simulink model "sampleModel548_pp_difftest"  (R2021a)
settings: Solver=VariableStepAuto  StartTime=0.0  StopTime=10.0  RelTol=1e-3
undefined symbols (not defined in the file or in its folder): DiscIntNeverNeededParam, Newton, Raphson
libraries: simulink x55, pid_lib x8
(part 2 of 2)

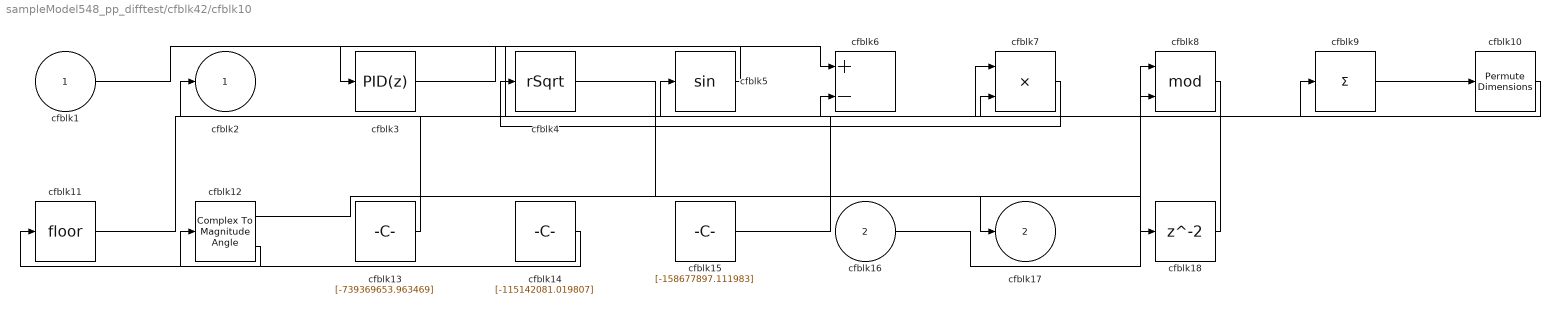
== system sampleModel548_pp_difftest/cfblk42/cfblk10 ==
  cfblk1 : Inport
  cfblk16 : Inport  Port=2
  cfblk10 : PermuteDimensions
  cfblk11 : Rounding
  cfblk12 : ComplexToMagnitudeAngle
  cfblk13 : Constant  Value=[-739369653.963469]  SampleTime=1
  cfblk14 : Constant  Value=[-115142081.019807]  SampleTime=1
  cfblk15 : Constant  Value=[-158677897.111983]  SampleTime=1
  cfblk18 : Delay  SampleTime=1
  cfblk3 : pid_lib/PID Controller  Controller=PID  Form=Parallel  TimeDomain=Discrete-time  UseExternalTs=off  SampleTime=1  IntegratorMethod=Forward Euler  FilterMethod=Forward Euler  ControllerParametersSource=internal  P=1  I=1  D=0  UseFilter=on  N=100  TunerSelectOption=Transfer Function Based (PID Tuner App)  InitialConditionSource=internal  InitialConditionForIntegrator=0  InitialConditionForFilter=0  DifferentiatorICPrevScaledInput=0  ExternalReset=none  TrackingMode=off  Kt=1  LimitOutput=off  SatLimitsSource=internal  UpperSaturationLimit=inf  LowerSaturationLimit=-inf  LinearizeAsGain=off  AntiWindupMode=none  Kb=1  POutMin=[]  POutMax=[]  IOutMin=[]  IOutMax=[]  DOutMin=[]  DOutMax=[]  NOutMin=[]  NOutMax=[]  SumOutMin=[]  SumOutMax=[]  SaturationOutMin=[]  SaturationOutMax=[]  PParamMin=[]  PParamMax=[]  IParamMin=[]  IParamMax=[]  DParamMin=[]  DParamMax=[]  NParamMin=[]  NParamMax=[]  KbParamMin=[]  KbParamMax=[]  KtParamMin=[]  KtParamMax=[]  KbOutMin=[]  KbOutMax=[]  KtOutMin=[]  KtOutMax=[]  IntegratorOutMin=[]  IntegratorOutMax=[]  FilterOutMin=[]  FilterOutMax=[]  SumI1OutMin=[]  SumI1OutMax=[]  SumI2OutMin=[]  SumI2OutMax=[]  SumI3OutMin=[]  SumI3OutMax=[]  SumI4OutMin=[]  SumI4OutMax=[]  SumDOutMin=[]  SumDOutMax=[]  DifferentiatorOutMin=[]  DifferentiatorOutMax=[]  FilterDiffOutCoefMin=[]  FilterDiffOutCoefMax=[]  ReciprocalOutMin=[]  ReciprocalOutMax=[]  SumDenOutMin=[]  SumDenOutMax=[]  SumNumOutMin=[]  SumNumOutMax=[]  DivideOutMin=[]  DivideOutMax=[]  UdiffTsProdOutMin=[]  UdiffTsProdOutMax=[]  NTsProdOutMin=[]  NTsProdOutMax=[]  UintegralTsProdOutMin=[]  UintegralTsProdOutMax=[]  UngainTsProdOutMin=[]  UngainTsProdOutMax=[]  IntegratorContinuousStateAttributes=''  IntegratorStateMustResolveToSignalObject=off  IntegratorRTWStateStorageClass=Auto  FilterContinuousStateAttributes=''  FilterStateMustResolveToSignalObject=off  FilterRTWStateStorageClass=Auto  ParallelPVariant=InternalParameters  IdealPVariant=Disabled  IVariant=InternalParameters  DVariant=InternalParameters  IntegratorVariant=Discrete  SatVariant=Disabled  AWVariant=Passthrough  PCopyVariant=Disabled  TRVariant=Disabled  FdbkBlocksVariant=Forward  IdealPFdbkVariant=Disabled  SatFdbkVariant=Disabled  DerivativeFilterVariant=ForwardEulerFilter  NVariant=InternalParameters  NCopyVariant=Disabled  FilterICVariant=InternalICsFilter  IntegratorICVariant=InternalICs  ExternalResetVariant=Disabled  TRSumVariant=Passthrough  SumFdbkVariant=Disabled  SumVariant=Sum_PID  TsampFilterVariant=InternalTs  TsampNgainVariant=Passthrough  TsampIntegralVariant=Passthrough  ExternalSaturationOutDataTypeStr=Inherit: Same as second input
  cfblk4 : Sqrt  Operator=rSqrt  AlgorithmType=Newton-Raphson  SaturateOnIntegerOverflow=on
  cfblk5 : Trigonometry
  cfblk6 : Sum  Inputs=+-
  cfblk7 : Product  Inputs=**
  cfblk8 : Math  Operator=mod  SaturateOnIntegerOverflow=on
  cfblk9 : Sum  Inputs=+
  cfblk2 : Outport
  cfblk17 : Outport  Port=2
  wires:
  cfblk12/1 -> cfblk17/1
  cfblk16/1 -> cfblk8/1
  cfblk14/1 -> cfblk12/1
  cfblk12/2 -> cfblk11/1
  cfblk13/1 -> cfblk2/1
  cfblk10/1 -> cfblk8/2
  cfblk1/1 -> cfblk7/2
  cfblk7/1 -> cfblk4/1
  cfblk15/1 -> cfblk9/1
  cfblk9/1 -> cfblk10/1
  cfblk11/1 -> cfblk5/1
  cfblk5/1 -> cfblk3/1
  cfblk3/1 -> cfblk6/1
  cfblk8/1 -> cfblk6/2
  cfblk4/1 -> cfblk18/1
  cfblk18/1 -> cfblk7/1

== system sampleModel548_pp_difftest/cfblk42/cfblk11 ==
  cfblk1 : Inport
  cfblk12 : Inport  Port=2
  cfblk13 : Inport  Port=3
  cfblk14 : Inport  Port=4
  cfblk15 : Inport  Port=5
  cfblk16 : Inport  Port=6
  cfblk10 : simulink/Math Operations/MinMax Running Resettable  Function=min  vinit=0.0
  cfblk11 : Constant  Value=[-708858344.222618]  SampleTime=1
  cfblk3 : DiscreteStateSpace
  cfblk4 : DiscreteIntegrator  ICPrevOutput=DiscIntNeverNeededParam  ICPrevScaledInput=DiscIntNeverNeededParam
  cfblk5 : UnitDelay  HasFrameUpgradeWarning=on
  cfblk6 : Delay  SampleTime=1
  cfblk7 : Sum  Inputs=-+
  cfblk8 : ComplexToMagnitudeAngle
  cfblk9 : ComplexToRealImag
  cfblk2 : Outport
  wires:
  cfblk15/1 -> cfblk5/1
  cfblk9/1 -> cfblk10/1
  cfblk3/1 -> cfblk7/1
  cfblk13/1 -> cfblk9/1
  cfblk7/1 -> cfblk2/1
  cfblk5/1 -> cfblk10/2
  cfblk6/1 -> cfblk8/1
  cfblk10/1 -> cfblk7/2
  cfblk1/1 -> cfblk6/1
  cfblk9/2 -> cfblk4/1
  cfblk4/1 -> cfblk3/1

== system sampleModel548_pp_difftest/cfblk42/cfblk8 ==
  cfblk1 : Inport
  cfblk11 : Inport  Port=2
  cfblk12 : Inport  Port=3
  cfblk13 : Inport  Port=4
  cfblk14 : Inport  Port=5
  cfblk10 : Constant  Value=[202416923.947961]  SampleTime=1
  cfblk17 : Delay  SampleTime=1
  cfblk3 : Delay  DelayLengthSource=Input port  SampleTime=1
      settings: InputPortMap=u0,p1
  cfblk4 : simulink/Discrete/Difference  ICPrevInput=0.0  OutMin=[]  OutMax=[]  OutDataTypeStr=Inherit: Inherit via back propagation  OutDataType=fixdt(1, 16)  OutScaling=2^-10  DoSatur=off
  cfblk5 : UnitDelay  HasFrameUpgradeWarning=on
  cfblk6 : MinMax
  cfblk7 : UnaryMinus
  cfblk8 : DotProduct  InputSameDT=on  OutDataTypeStr=Inherit: Inherit via internal rule
  cfblk9 : Constant  Value=[-329113681.085165]  SampleTime=1
  cfblk2 : Outport
  cfblk15 : Outport  Port=2
  cfblk16 : Outport  Port=3
  wires:
  cfblk10/1 -> cfblk5/1
  cfblk4/1 -> cfblk2/1
  cfblk11/1 -> cfblk7/1
  cfblk12/1 -> cfblk15/1
  cfblk13/1 -> cfblk8/1
  cfblk5/1 -> cfblk16/1
  cfblk6/1 -> cfblk8/2
  cfblk9/1 -> cfblk3/1
  cfblk7/1 -> cfblk4/1
  cfblk1/1 -> cfblk3/2
  cfblk8/1 -> cfblk17/1
  cfblk17/1 -> cfblk6/1

== system sampleModel548_pp_difftest/cfblk42/cfblk9 ==
  cfblk1 : Inport
  cfblk6 : Inport  Port=2
  cfblk7 : Inport  Port=3
  cfblk3 : simulink/Discrete/Transfer Fcn Lead or Lag  PoleZ=0.95  ZeroZ=0.75  ICPrevOutput=0.0  ICPrevInput=0.0  DoSatur=off
      settings: SourceProductBaseCode=SL
  cfblk4 : Delay  DelayLengthSource=Input port  SampleTime=1
      settings: InputPortMap=u0,p1
  cfblk5 : Constant  Value=[-290514364.300051]  SampleTime=1
  cfblk8 : Delay  SampleTime=1
  cfblk2 : Outport
  wires:
  cfblk6/1 -> cfblk2/1
  cfblk7/1 -> cfblk4/1
  cfblk3/1 -> cfblk4/2
  cfblk4/1 -> cfblk8/1
  cfblk8/1 -> cfblk3/1

== system sampleModel548_pp_difftest/cfblk43/cfblk10 ==
  cfblk1 : Inport
  cfblk7 : Inport  Port=2
  cfblk8 : Inport  Port=3
  cfblk9 : Inport  Port=4
  cfblk10 : Inport  Port=5
  cfblk11 : Inport  Port=6
  cfblk12 : Inport  Port=7
  cfblk13 : Delay  SampleTime=1
  cfblk3 : Polyval  Coefs=[ +2.081618890e-019, -1.441693666e-014, +4.719686976e-010, -8.536869453e-006, +1.621573104e-001, -8.087801117e+001 ]
  cfblk4 : PermuteDimensions
  cfblk5 : ComplexToRealImag
  cfblk6 : Constant  Value=[-161923909.561596]  SampleTime=1
  cfblk2 : Outport
  wires:
  cfblk1/1 -> cfblk2/1
  cfblk3/1 -> cfblk5/1
  cfblk7/1 -> cfblk4/1
  cfblk5/1 -> cfblk13/1
  cfblk13/1 -> cfblk3/1

== system sampleModel548_pp_difftest/cfblk43/cfblk11 ==
  cfblk1 : Inport
  cfblk14 : Inport  Port=2
  cfblk15 : Inport  Port=3
  cfblk16 : Inport  Port=4
  cfblk10 : ComplexToRealImag
  cfblk11 : Product  Inputs=*
  cfblk12 : Sqrt  Operator=rSqrt  AlgorithmType=Newton-Raphson  SaturateOnIntegerOverflow=on
  cfblk13 : Math  Operator=mod  SaturateOnIntegerOverflow=on
  cfblk3 : DiscreteStateSpace
  cfblk4 : pid_lib/PID Controller (2DOF)  Controller=PID  Form=Parallel  TimeDomain=Discrete-time  UseExternalTs=off  SampleTime=1  IntegratorMethod=Forward Euler  FilterMethod=Forward Euler  ControllerParametersSource=internal  P=1  I=1  D=0  UseFilter=on  N=100  b=1  c=1  TunerSelectOption=Transfer Function Based (PID Tuner App)  InitialConditionSource=internal  InitialConditionForIntegrator=0  InitialConditionForFilter=0  DifferentiatorICPrevScaledInput=0  ExternalReset=none  TrackingMode=off  Kt=1  LimitOutput=off  SatLimitsSource=internal  UpperSaturationLimit=inf  LowerSaturationLimit=-inf  LinearizeAsGain=off  AntiWindupMode=none  Kb=1  POutMin=[]  POutMax=[]  IOutMin=[]  IOutMax=[]  DOutMin=[]  DOutMax=[]  NOutMin=[]  NOutMax=[]  bOutMin=[]  bOutMax=[]  cOutMin=[]  cOutMax=[]  SumOutMin=[]  SumOutMax=[]  SaturationOutMin=[]  SaturationOutMax=[]  PParamMin=[]  PParamMax=[]  IParamMin=[]  IParamMax=[]  DParamMin=[]  DParamMax=[]  NParamMin=[]  NParamMax=[]  bParamMin=[]  bParamMax=[]  cParamMin=[]  cParamMax=[]  KbParamMin=[]  KbParamMax=[]  KtParamMin=[]  KtParamMax=[]  KbOutMin=[]  KbOutMax=[]  KtOutMin=[]  KtOutMax=[]  IntegratorOutMin=[]  IntegratorOutMax=[]  FilterOutMin=[]  FilterOutMax=[]  SumI1OutMin=[]  SumI1OutMax=[]  SumI2OutMin=[]  SumI2OutMax=[]  SumI3OutMin=[]  SumI3OutMax=[]  SumI4OutMin=[]  SumI4OutMax=[]  SumDOutMin=[]  SumDOutMax=[]  Sum1OutMin=[]  Sum1OutMax=[]  Sum2OutMin=[]  Sum2OutMax=[]  Sum3OutMin=[]  Sum3OutMax=[]  DifferentiatorOutMin=[]  DifferentiatorOutMax=[]  FilterDiffOutCoefMin=[]  FilterDiffOutCoefMax=[]  ReciprocalOutMin=[]  ReciprocalOutMax=[]  SumDenOutMin=[]  SumDenOutMax=[]  SumNumOutMin=[]  SumNumOutMax=[]  DivideOutMin=[]  DivideOutMax=[]  UdiffTsProdOutMin=[]  UdiffTsProdOutMax=[]  NTsProdOutMin=[]  NTsProdOutMax=[]  UintegralTsProdOutMin=[]  UintegralTsProdOutMax=[]  UngainTsProdOutMin=[]  UngainTsProdOutMax=[]  IntegratorContinuousStateAttributes=''  IntegratorStateMustResolveToSignalObject=off  IntegratorRTWStateStorageClass=Auto  FilterContinuousStateAttributes=''  FilterStateMustResolveToSignalObject=off  FilterRTWStateStorageClass=Auto  ParallelPVariant=InternalParameters  IdealPVariant=Disabled  IVariant=InternalParameters  DVariant=InternalParameters  bVariant=InternalParameters  cVariant=InternalParameters  IntegratorVariant=Discrete  SatVariant=Disabled  AWVariant=Passthrough  PCopyVariant=Disabled  TRVariant=Disabled  FdbkBlocksVariant=Forward  IdealPFdbkVariant=Disabled  SatFdbkVariant=Disabled  DerivativeFilterVariant=ForwardEulerFilter  NVariant=InternalParameters  NCopyVariant=Disabled  FilterICVariant=InternalICsFilter  IntegratorICVariant=InternalICs  ExternalResetVariant=Disabled  TRSumVariant=Passthrough  SumFdbkVariant=Disabled  SumVariant=Sum_PID  TsampFilterVariant=InternalTs  TsampNgainVariant=Passthrough  TsampIntegralVariant=Passthrough  ExternalSaturationOutDataTypeStr=Inherit: Same as second input
      settings: SourceProductBaseCode=SL
  cfblk5 : simulink/Discrete/Tapped Delay  vinit=0.0  samptime=-1  NumDelays=1  DelayOrder=Oldest  includeCurrent=off
  cfblk6 : DiscreteZeroPole  Poles=[0 0.5]  Gain=1
  cfblk7 : Sum  Inputs=+
  cfblk8 : simulink/Math Operations/Slider Gain  gain=1  low=0  high=2
  cfblk9 : Bias  Bias=[-967330552.084778]
  cfblk2 : Outport
  cfblk17 : Outport  Port=2
  wires:
  cfblk10/1 -> cfblk17/1
  cfblk13/1 -> cfblk3/1
  cfblk12/1 -> cfblk4/1
  cfblk4/1 -> cfblk8/1
  cfblk6/1 -> cfblk4/2
  cfblk5/1 -> cfblk7/1
  cfblk7/1 -> cfblk6/1
  cfblk8/1 -> cfblk2/1
  cfblk10/2 -> cfblk5/1
  cfblk15/1 -> cfblk9/1
  cfblk9/1 -> cfblk13/1
  cfblk16/1 -> cfblk11/1
  cfblk11/1 -> cfblk10/1
  cfblk14/1 -> cfblk13/2
  cfblk3/1 -> cfblk12/1

== system sampleModel548_pp_difftest/cfblk43/cfblk15 ==
  cfblk1 : Inport
  cfblk10 : Inport  Port=2
  cfblk11 : Inport  Port=3
  Action Port : ActionPort  ActionPortLabel=if(u1 >= 0)
  cfblk12 : Delay
  cfblk3 : Delay  DelayLengthSource=Input port
      settings: InputPortMap=u0,p1
  cfblk4 : Sum  Inputs=+
  cfblk5 : Sum  Inputs=+-
  cfblk6 : Product  Inputs=**
  cfblk7 : Product
  cfblk8 : Constant  Value=[-890965231.950581]  SampleTime=1
  cfblk9 : Constant  Value=[-398540983.405424]  SampleTime=1
  cfblk2 : Outport
  wires:
  cfblk3/1 -> cfblk7/1
  cfblk8/1 -> cfblk5/1
  cfblk4/1 -> cfblk6/1
  cfblk10/1 -> cfblk7/2
  cfblk9/1 -> cfblk6/2
  cfblk1/1 -> cfblk2/1
  cfblk7/1 -> cfblk4/1
  cfblk11/1 -> cfblk5/2
  cfblk5/1 -> cfblk3/2
  cfblk6/1 -> cfblk12/1
  cfblk12/1 -> cfblk3/1

== system sampleModel548_pp_difftest/cfblk43/cfblk16 ==
  cfblk1 : Inport
  cfblk9 : Inport  Port=2
  Action Port : ActionPort  ActionPortLabel=else
  cfblk12 : Delay
  cfblk3 : simulink/Discrete/Tapped Delay  vinit=0.0  samptime=-1  NumDelays=1  DelayOrder=Oldest  includeCurrent=off
  cfblk4 : DiscreteZeroPole  Poles=[0 0.5]  Gain=1  SampleTime=-1
  cfblk5 : DiscreteFilter
  cfblk6 : simulink/Discrete/Transfer Fcn Real Zero  ZeroZ=0.75  ICPrevInput=0.0  DoSatur=off
      settings: SourceProductBaseCode=SL
  cfblk7 : Assignment  DiagnosticForDimensions=Warning  IndexOptions=Index vector (dialog)  Indices=1  OutputSizes=1
  cfblk8 : Constant  Value=[544364623.846351]  SampleTime=1
  cfblk2 : Outport
  cfblk10 : Outport  Port=2
  cfblk11 : Outport  Port=3
  wires:
  cfblk8/1 -> cfblk10/1
  cfblk7/1 -> cfblk4/1
  cfblk5/1 -> cfblk2/1
  cfblk4/1 -> cfblk11/1, cfblk5/1
  cfblk9/1 -> cfblk7/1
  cfblk1/1 -> cfblk7/2
  cfblk3/1 -> cfblk6/1
  cfblk6/1 -> cfblk12/1
  cfblk12/1 -> cfblk3/1

== system sampleModel548_pp_difftest/cfblk44/cfblk9 ==
  cfblk1 : Inport
  cfblk11 : Inport  Port=2
  cfblk10 : Constant  Value=[613050272.932422]  SampleTime=1
  cfblk3 : DiscreteZeroPole  Poles=[0 0.5]  Gain=1
  cfblk4 : DiscreteIntegrator  ICPrevOutput=DiscIntNeverNeededParam  ICPrevScaledInput=DiscIntNeverNeededParam
  cfblk5 : UnitDelay  HasFrameUpgradeWarning=on
  cfblk6 : Sin  TimeSource=Use external signal  SampleTime=0
  cfblk7 : Abs
  cfblk8 : simulink/Math Operations/MinMax Running Resettable  Function=min  vinit=0.0
  cfblk9 : simulink/Math Operations/Slider Gain  gain=1  low=0  high=2
  cfblk2 : Outport
  cfblk12 : Outport  Port=2
  wires:
  cfblk4/1 -> cfblk7/1
  cfblk9/1 -> cfblk5/1
  cfblk8/1 -> cfblk12/1
  cfblk11/1 -> cfblk2/1
  cfblk3/1 -> cfblk6/1
  cfblk6/1 -> cfblk8/1
  cfblk5/1 -> cfblk4/1
  cfblk1/1 -> cfblk8/2
  cfblk7/1 -> cfblk3/1
  cfblk10/1 -> cfblk9/1

== system sampleModel548_pp_difftest/cfblk45/cfblk11 ==
  cfblk1 : Inport
  cfblk9 : Inport  Port=2
  cfblk10 : Inport  Port=3
  cfblk11 : Inport  Port=4
  cfblk3 : simulink/Discrete/Difference  ICPrevInput=0.0  OutMin=[]  OutMax=[]  OutDataTypeStr=Inherit: Inherit via back propagation  OutDataType=fixdt(1, 16)  OutScaling=2^-10  DoSatur=off
  cfblk4 : DiscreteFilter  SampleTime=1
  cfblk5 : Gain  Gain=[-789682304.359005]
  cfblk6 : Product  Inputs=**
  cfblk7 : Bias  Bias=[363494201.549703]
  cfblk8 : Polyval  Coefs=[ +2.081618890e-019, -1.441693666e-014, +4.719686976e-010, -8.536869453e-006, +1.621573104e-001, -8.087801117e+001 ]
  cfblk2 : Outport
  cfblk12 : Outport  Port=2
  cfblk13 : Outport  Port=3
  cfblk14 : Outport  Port=4
  cfblk15 : Outport  Port=5
  wires:
  cfblk11/1 -> cfblk14/1, cfblk5/1
  cfblk3/1 -> cfblk8/1, cfblk13/1
  cfblk1/1 -> cfblk6/1
  cfblk8/1 -> cfblk12/1
  cfblk7/1 -> cfblk6/2
  cfblk9/1 -> cfblk2/1
  cfblk10/1 -> cfblk4/1
  cfblk6/1 -> cfblk3/1
  cfblk5/1 -> cfblk15/1
  cfblk4/1 -> cfblk7/1

== system sampleModel548_pp_difftest/cfblk45/cfblk12 ==
  cfblk1 : Inport
  cfblk11 : Delay  SampleTime=1
  cfblk3 : Delay  SampleTime=1
  cfblk4 : DiscreteFilter  SampleTime=1
  cfblk5 : Sin  TimeSource=Use external signal  SampleTime=0
  cfblk6 : Math  Operator=pow  SaturateOnIntegerOverflow=on
  cfblk7 : Product  Inputs=**
  cfblk8 : Polyval  Coefs=[ +2.081618890e-019, -1.441693666e-014, +4.719686976e-010, -8.536869453e-006, +1.621573104e-001, -8.087801117e+001 ]
  cfblk9 : Constant  Value=[385539584.966270]  SampleTime=1
  cfblk2 : Outport
  cfblk10 : Outport  Port=2
  wires:
  cfblk1/1 -> cfblk8/1, cfblk4/1
  cfblk9/1 -> cfblk5/1
  cfblk4/1 -> cfblk2/1
  cfblk5/1 -> cfblk6/1, cfblk6/2
  cfblk6/1 -> cfblk7/1
  cfblk3/1 -> cfblk7/2
  cfblk8/1 -> cfblk10/1
  cfblk7/1 -> cfblk11/1
  cfblk11/1 -> cfblk3/1

== system sampleModel548_pp_difftest/cfblk45/cfblk13 ==
  cfblk1 : Inport
  cfblk9 : Inport  Port=2
  cfblk3 : simulink/Discrete/Tapped Delay  vinit=0.0  samptime=-1  NumDelays=1  DelayOrder=Oldest  includeCurrent=off
  cfblk4 : simulink/Discrete/Transfer Fcn First Order  PoleZ=0.95  ICPrevOutput=0.0  DoSatur=off
  cfblk5 : simulink/Math Operations/Slider Gain  gain=1  low=0  high=2
  cfblk6 : Sqrt  Operator=rSqrt  AlgorithmType=Newton-Raphson  SaturateOnIntegerOverflow=on
  cfblk7 : Constant  Value=[-501479578.352141]  SampleTime=1
  cfblk8 : Constant  Value=[-19645125.250562]  SampleTime=1
  cfblk2 : Outport
  wires:
  cfblk3/1 -> cfblk5/1
  cfblk7/1 -> cfblk4/1
  cfblk1/1 -> cfblk3/1
  cfblk4/1 -> cfblk2/1
  cfblk5/1 -> cfblk6/1

== system sampleModel548_pp_difftest/cfblk46/cfblk12 ==
  cfblk1 : Inport
  cfblk11 : Inport  Port=2
  cfblk12 : Inport  Port=3
  cfblk13 : Inport  Port=4
  cfblk14 : Inport  Port=5
  cfblk10 : Sum
  cfblk3 : Delay  ShowEnablePort=on  SampleTime=1
      settings: InputPortMap=u0,e6
  cfblk4 : simulink/Discrete/Tapped Delay  vinit=0.0  samptime=-1  NumDelays=1  DelayOrder=Oldest  includeCurrent=off
  cfblk5 : Sum  Inputs=|++
  cfblk6 : Squeeze
  cfblk7 : Polyval  Coefs=[ +2.081618890e-019, -1.441693666e-014, +4.719686976e-010, -8.536869453e-006, +1.621573104e-001, -8.087801117e+001 ]
  cfblk8 : ComplexToRealImag
  cfblk9 : Gain  Gain=[-355568731.986188]
  cfblk2 : Outport
  cfblk15 : Outport  Port=2
  cfblk16 : Outport  Port=3
  wires:
  cfblk1/1 -> cfblk9/1
  cfblk6/1 -> cfblk7/1
  cfblk8/1 -> cfblk2/1
  cfblk12/1 -> cfblk10/1
  cfblk8/2 -> cfblk15/1
  cfblk13/1 -> cfblk4/1
  cfblk4/1 -> cfblk8/1
  cfblk7/1 -> cfblk5/1
  cfblk14/1 -> cfblk3/1
  cfblk9/1 -> cfblk10/2
  cfblk10/1 -> cfblk6/1
  cfblk3/1 -> cfblk5/2
  cfblk5/1 -> cfblk16/1
  cfblk11/1 -> cfblk3/2

== system sampleModel548_pp_difftest/cfblk47/cfblk11 ==
  cfblk1 : Inport
  cfblk7 : Inport  Port=2
  cfblk8 : Inport  Port=3
  cfblk9 : Inport  Port=4
  cfblk3 : DiscreteStateSpace
  cfblk4 : Sum  Inputs=-+
  cfblk5 : Math  Operator=log10  SaturateOnIntegerOverflow=on
  cfblk6 : Constant  Value=[-513662995.683131]  SampleTime=1
  cfblk2 : Outport
  wires:
  cfblk5/1 -> cfblk2/1
  cfblk9/1 -> cfblk3/1
  cfblk6/1 -> cfblk4/1
  cfblk1/1 -> cfblk4/2
  cfblk8/1 -> cfblk5/1

== system sampleModel548_pp_difftest/cfblk47/cfblk12 ==
  cfblk1 : Inport
  cfblk10 : Inport  Port=2
  cfblk11 : Inport  Port=3
  cfblk12 : Inport  Port=4
  cfblk16 : Delay  SampleTime=1
  cfblk3 : DiscreteStateSpace
  cfblk4 : DiscreteFilter  SampleTime=1
  cfblk5 : simulink/Discrete/Transfer Fcn Real Zero  ZeroZ=0.75  ICPrevInput=0.0  DoSatur=off
      settings: SourceProductBaseCode=SL
  cfblk6 : Assignment  DiagnosticForDimensions=Warning  IndexOptions=Index vector (dialog)  Indices=1  OutputSizes=1
  cfblk7 : UnaryMinus
  cfblk8 : simulink/Math Operations/MinMax Running Resettable  Function=min  vinit=0.0
  cfblk9 : Constant  Value=[195595849.733871]  SampleTime=1
  cfblk2 : Outport
  cfblk13 : Outport  Port=2
  cfblk14 : Outport  Port=3
  cfblk15 : Outport  Port=4
  wires:
  cfblk10/1 -> cfblk7/1
  cfblk12/1 -> cfblk6/1
  cfblk9/1 -> cfblk4/1
  cfblk6/1 -> cfblk13/1
  cfblk11/1 -> cfblk8/1
  cfblk1/1 -> cfblk14/1
  cfblk3/1 -> cfblk8/2, cfblk6/2
  cfblk7/1 -> cfblk2/1
  cfblk5/1 -> cfblk15/1
  cfblk4/1 -> cfblk5/1
  cfblk8/1 -> cfblk16/1
  cfblk16/1 -> cfblk3/1

== system sampleModel548_pp_difftest/cfblk48/cfblk12 ==
  cfblk1 : Inport
  cfblk10 : Inport  Port=2
  Action Port : ActionPort  ActionPortLabel=if(u1 >= 0)
  cfblk3 : simulink/Discrete/Transfer Fcn Lead or Lag  PoleZ=0.95  ZeroZ=0.75  ICPrevOutput=0.0  ICPrevInput=0.0  DoSatur=off
      settings: SourceProductBaseCode=SL
  cfblk4 : Delay
  cfblk5 : simulink/Discrete/Transfer Fcn Real Zero  ZeroZ=0.75  ICPrevInput=0.0  DoSatur=off
      settings: SourceProductBaseCode=SL
  cfblk6 : Sum  Inputs=+-
  cfblk7 : Abs
  cfblk8 : Constant  Value=[125327127.565151]  SampleTime=1
  cfblk9 : Constant  Value=[-877843957.343057]  SampleTime=1
  cfblk2 : Outport
  wires:
  cfblk10/1 -> cfblk5/1
  cfblk9/1 -> cfblk2/1
  cfblk4/1 -> cfblk6/1
  cfblk8/1 -> cfblk6/2
  cfblk1/1 -> cfblk7/1
  cfblk3/1 -> cfblk4/1
  cfblk5/1 -> cfblk3/1

== system sampleModel548_pp_difftest/cfblk48/cfblk13 ==
  cfblk1 : Inport
  cfblk12 : Inport  Port=2
  cfblk13 : Inport  Port=3
  Action Port : ActionPort  ActionPortLabel=else
  cfblk10 : Constant  Value=[696700765.122219]  SampleTime=1
  cfblk11 : Constant  Value=[151616286.059709]  SampleTime=1
  cfblk14 : Delay
  cfblk3 : simulink/Discrete/Transfer Fcn Real Zero  ZeroZ=0.75  ICPrevInput=0.0  DoSatur=off
      settings: SourceProductBaseCode=SL
  cfblk4 : simulink/Discrete/Transfer Fcn First Order  PoleZ=0.95  ICPrevOutput=0.0  DoSatur=off
  cfblk5 : Delay  ShowEnablePort=on
      settings: InputPortMap=u0,e6
  cfblk6 : Abs
  cfblk7 : Sqrt  Operator=rSqrt  AlgorithmType=Newton-Raphson  SaturateOnIntegerOverflow=on
  cfblk8 : simulink/Math Operations/MinMax Running Resettable  Function=min  vinit=0.0
  cfblk9 : Constant  Value=[700965549.820929]  SampleTime=1
  cfblk2 : Outport
  wires:
  cfblk5/1 -> cfblk7/1
  cfblk3/1 -> cfblk8/1
  cfblk11/1 -> cfblk4/1
  cfblk4/1 -> cfblk6/1
  cfblk10/1 -> cfblk2/1
  cfblk13/1 -> cfblk3/1
  cfblk6/1 -> cfblk5/2
  cfblk9/1 -> cfblk8/2
  cfblk7/1 -> cfblk14/1
  cfblk14/1 -> cfblk5/1

== system sampleModel548_pp_difftest/cfblk48/cfblk6 ==
  cfblk1 : Inport
  cfblk11 : Inport  Port=2
  cfblk12 : Inport  Port=3
  cfblk13 : Inport  Port=4
  cfblk10 : Constant  Value=[-108899001.625536]  SampleTime=1
  cfblk3 : Delay  DelayLengthSource=Input port  SampleTime=1
      settings: InputPortMap=u0,p1
  cfblk4 : DiscreteZeroPole  Poles=[0 0.5]  Gain=1
  cfblk5 : simulink/Discrete/Tapped Delay  vinit=0.0  samptime=-1  NumDelays=1  DelayOrder=Oldest  includeCurrent=off
  cfblk6 : simulink/Discrete/Difference  ICPrevInput=0.0  OutMin=[]  OutMax=[]  OutDataTypeStr=Inherit: Inherit via back propagation  OutDataType=fixdt(1, 16)  OutScaling=2^-10  DoSatur=off
  cfblk7 : DiscreteFir  SampleTime=1
  cfblk8 : simulink/Math Operations/Slider Gain  gain=1  low=0  high=2
  cfblk9 : DotProduct  InputSameDT=on  OutDataTypeStr=Inherit: Inherit via internal rule
  cfblk2 : Outport
  wires:
  cfblk10/1 -> cfblk9/1
  cfblk1/1 -> cfblk4/1
  cfblk7/1 -> cfblk3/1
  cfblk9/1 -> cfblk2/1
  cfblk11/1 -> cfblk8/1
  cfblk13/1 -> cfblk6/1
  cfblk5/1 -> cfblk9/2
  cfblk4/1 -> cfblk3/2
  cfblk3/1 -> cfblk5/1
  cfblk12/1 -> cfblk7/1

== system sampleModel548_pp_difftest/cfblk48/cfblk7 ==
  cfblk1 : Inport
  cfblk8 : Inport  Port=2
  cfblk3 : Squeeze
  cfblk4 : MinMax  Inputs=3
  cfblk5 : PermuteDimensions
  cfblk6 : Constant  Value=[478490921.167015]  SampleTime=1
  cfblk7 : Constant  Value=[891051676.802070]  SampleTime=1
  cfblk2 : Outport
  wires:
  cfblk5/1 -> cfblk4/1
  cfblk4/1 -> cfblk2/1
  cfblk6/1 -> cfblk3/1
  cfblk3/1 -> cfblk5/1
  cfblk8/1 -> cfblk4/2
  cfblk1/1 -> cfblk4/3

== system sampleModel548_pp_difftest/cfblk48/cfblk8 ==
  cfblk1 : Inport
  cfblk10 : Inport  Port=2
  cfblk11 : Inport  Port=3
  cfblk12 : Inport  Port=4
  cfblk13 : Inport  Port=5
  cfblk15 : Delay  SampleTime=1
  cfblk3 : Delay  SampleTime=1
  cfblk4 : DiscreteZeroPole  Poles=[0 0.5]  Gain=1
  cfblk5 : Sin  TimeSource=Use external signal  SampleTime=0
  cfblk6 : Squeeze
  cfblk7 : Sin  TimeSource=Use external signal  SampleTime=0
  cfblk8 : Rounding
  cfblk9 : Constant  Value=[-379912177.321118]  SampleTime=1
  cfblk2 : Outport
  cfblk14 : Outport  Port=2
  wires:
  cfblk3/1 -> cfblk7/1
  cfblk8/1 -> cfblk6/1
  cfblk10/1 -> cfblk3/1
  cfblk5/1 -> cfblk14/1
  cfblk12/1 -> cfblk5/1
  cfblk1/1 -> cfblk2/1
  cfblk4/1 -> cfblk8/1
  cfblk6/1 -> cfblk15/1
  cfblk15/1 -> cfblk4/1

== system sampleModel548_pp_difftest/cfblk48/cfblk9 ==
  cfblk1 : Inport
  cfblk12 : Inport  Port=2
  cfblk13 : Inport  Port=3
  cfblk10 : Bias  Bias=[78693443.823464]
  cfblk11 : Constant  Value=[-451602254.551171]  SampleTime=1
  cfblk3 : simulink/Discrete/Transfer Fcn First Order  PoleZ=0.95  ICPrevOutput=0.0  DoSatur=off
  cfblk4 : DiscreteFilter  SampleTime=1
  cfblk5 : Reshape
  cfblk6 : Squeeze
  cfblk7 : Math  Operator=rem  SaturateOnIntegerOverflow=on
  cfblk8 : Product  Inputs=*
  cfblk9 : Product  Inputs=*
  cfblk2 : Outport
  cfblk14 : Outport  Port=2
  wires:
  cfblk7/1 -> cfblk14/1
  cfblk9/1 -> cfblk7/1
  cfblk6/1 -> cfblk7/2
  cfblk8/1 -> cfblk4/1
  cfblk12/1 -> cfblk3/1
  cfblk13/1 -> cfblk5/1
  cfblk3/1 -> cfblk10/1
  cfblk5/1 -> cfblk8/1
  cfblk1/1 -> cfblk9/1
  cfblk10/1 -> cfblk2/1
  cfblk11/1 -> cfblk6/1

== system sampleModel548_pp_difftest/cfblk49/cfblk7 ==
  cfblk1 : Inport
  cfblk13 : Inport  Port=2
  cfblk14 : Inport  Port=3
  cfblk10 : Product
  cfblk11 : Sum  Inputs=+-
  cfblk12 : Sqrt  Operator=rSqrt  AlgorithmType=Newton-Raphson  SaturateOnIntegerOverflow=on
  cfblk16 : Delay  SampleTime=1
  cfblk3 : DiscreteTransferFcn  SampleTime=1
  cfblk4 : Delay  SampleTime=1
  cfblk5 : DiscreteZeroPole  Poles=[0 0.5]  Gain=1
  cfblk6 : Delay  SampleTime=1
  cfblk7 : Delay  DelayLengthSource=Input port  SampleTime=1
      settings: InputPortMap=u0,p1
  cfblk8 : Sum  Inputs=+
  cfblk9 : Trigonometry
  cfblk2 : Outport
  cfblk15 : Outport  Port=2
  wires:
  cfblk6/1 -> cfblk4/1
  cfblk4/1 -> cfblk11/1
  cfblk12/1 -> cfblk15/1
  cfblk9/1 -> cfblk2/1, cfblk16/1
  cfblk11/1 -> cfblk8/1
  cfblk13/1 -> cfblk3/1
  cfblk7/1 -> cfblk5/1
  cfblk5/1 -> cfblk6/1
  cfblk8/1 -> cfblk10/1
  cfblk1/1 -> cfblk11/2
  cfblk10/1 -> cfblk12/1, cfblk9/1
  cfblk3/1 -> cfblk7/1
  cfblk14/1 -> cfblk7/2
  cfblk16/1 -> cfblk10/2

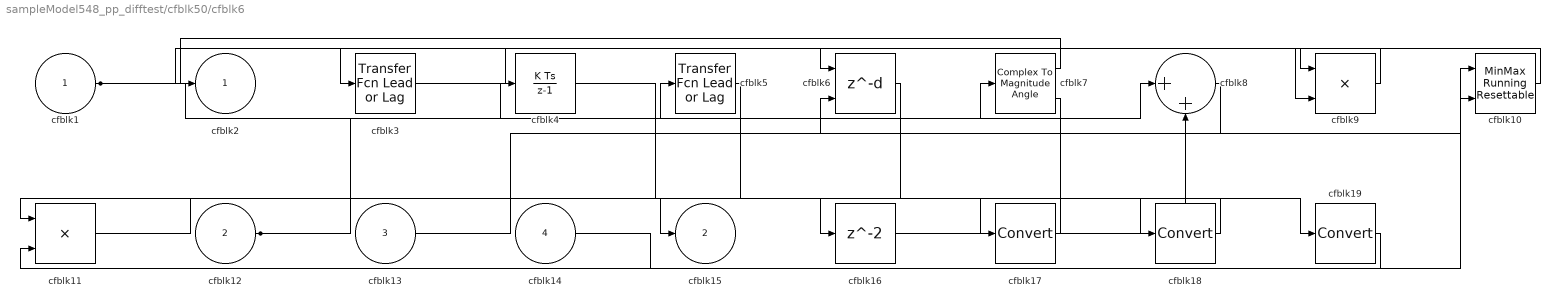
== system sampleModel548_pp_difftest/cfblk50/cfblk6 ==
  cfblk1 : Inport
  cfblk12 : Inport  Port=2
  cfblk13 : Inport  Port=3
  cfblk14 : Inport  Port=4
  cfblk10 : simulink/Math Operations/MinMax Running Resettable  Function=min  vinit=0.0
  cfblk11 : Product
  cfblk16 : Delay  SampleTime=1
  cfblk17 : DataTypeConversion
  cfblk18 : DataTypeConversion
  cfblk19 : DataTypeConversion
  cfblk3 : simulink/Discrete/Transfer Fcn Lead or Lag  PoleZ=0.95  ZeroZ=0.75  ICPrevOutput=0.0  ICPrevInput=0.0  DoSatur=off
      settings: SourceProductBaseCode=SL
  cfblk4 : DiscreteIntegrator  ICPrevOutput=DiscIntNeverNeededParam  ICPrevScaledInput=DiscIntNeverNeededParam
  cfblk5 : simulink/Discrete/Transfer Fcn Lead or Lag  PoleZ=0.95  ZeroZ=0.75  ICPrevOutput=0.0  ICPrevInput=0.0  DoSatur=off
      settings: SourceProductBaseCode=SL
  cfblk6 : Delay  DelayLengthSource=Input port  SampleTime=1
      settings: InputPortMap=u0,p1
  cfblk7 : ComplexToMagnitudeAngle
  cfblk8 : Sum  Inputs=|++
  cfblk9 : Product
  cfblk2 : Outport
  cfblk15 : Outport  Port=2
  wires:
  cfblk3/1 -> cfblk6/1
  cfblk1/1 -> cfblk8/1, cfblk9/2
  cfblk7/1 -> cfblk2/1
  cfblk5/1 -> cfblk15/1
  cfblk7/2 -> cfblk5/1
  cfblk14/1 -> cfblk10/1
  cfblk10/1 -> cfblk9/1
  cfblk13/1 -> cfblk10/2
  cfblk12/1 -> cfblk4/1, cfblk19/1
  cfblk8/1 -> cfblk6/2
  cfblk9/1 -> cfblk3/1
  cfblk6/1 -> cfblk16/1
  cfblk16/1 -> cfblk8/2
  cfblk11/1 -> cfblk17/1
  cfblk17/1 -> cfblk7/1
  cfblk4/1 -> cfblk18/1
  cfblk18/1 -> cfblk11/1
  cfblk19/1 -> cfblk11/2
